simulink model "PIDController"  (R2025b)
settings: Solver=FixedStepAuto  StartTime=0.0  StopTime=inf  FixedStep=.002  RelTol=1e-3
libraries: simulink x3
settings Model: Creator=ajax  LastModifiedBy=ajax

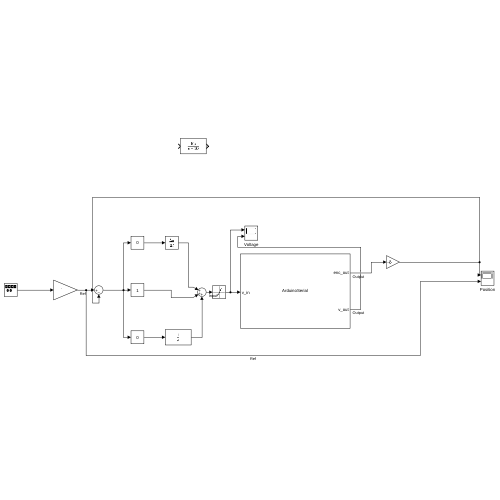
[thumbnail: Simulink's stored preview of the top-level diagram]
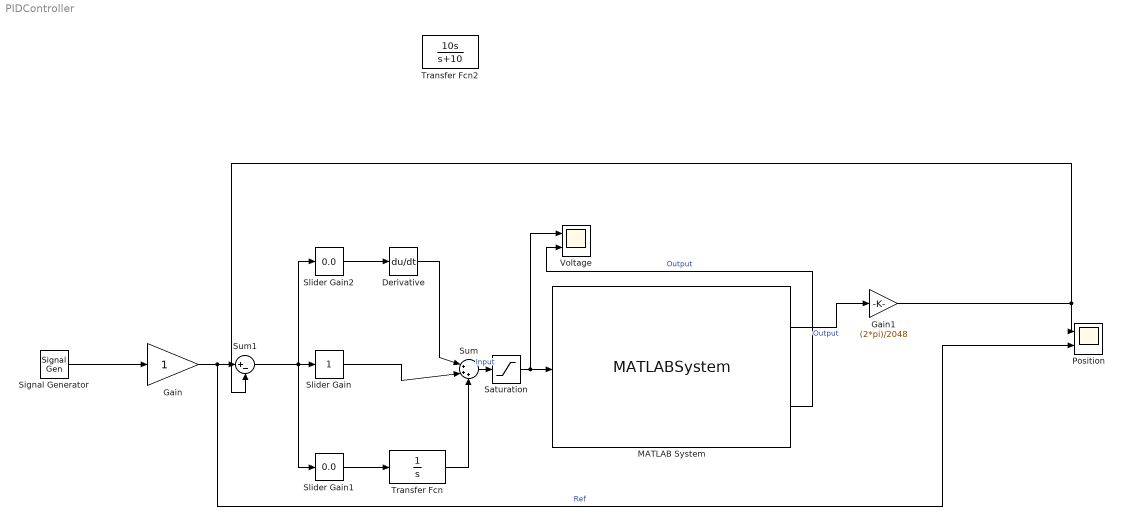
== system PIDController ==
  Derivative : Derivative
  Gain : Gain
  Gain1 : Gain  Gain=(2*pi)/2048
  MATLAB System : MATLABSystem  System=ArduinoSerial  COMPort=/dev/ttyACM0  BaudRate=115200  TimerPeriod=0.005  SimulateUsing=Interpreted execution
      mask Type: ArduinoSerial
  Position : Scope  NumInputPorts=2
      settings: ActiveDisplayYMinimum=-365.02359945676773  ActiveDisplayYMaximum=873.0296356104534
  Saturation : Saturate  UpperLimit=3  LowerLimit=-3
  Signal Generator : SignalGenerator  WaveForm=square  Frequency=.5
  Slider Gain : simulink/Math Operations/Slider Gain  gain=1  low=0  high=2
  Slider Gain1 : simulink/Math Operations/Slider Gain  gain=0.0  low=0  high=2
  Slider Gain2 : simulink/Math Operations/Slider Gain  gain=0.0  low=0  high=10
  Sum : Sum  Inputs=|+++
  Sum1 : Sum  Inputs=|+-
  Transfer Fcn : TransferFcn  Denominator=[1 0]
  Transfer Fcn2 : TransferFcn  Numerator=[10 0]  Denominator=[1 10]
  Voltage : Scope  NumInputPorts=2
      settings: ActiveDisplayYMinimum=-7.1806488970151925  ActiveDisplayYMaximum=7.8345844750588949
  wires:
  Slider Gain/1 -> Sum/2
  Slider Gain1/1 -> Transfer Fcn/1
  Transfer Fcn/1 -> Sum/3
  MATLAB System/1 -> Gain1/1  "Output"
  Gain/1 -> Position/2, Sum1/1  "Ref"
  MATLAB System/2 -> Voltage/2  "Output"
  Sum1/1 -> Slider Gain2/1, Slider Gain1/1, Slider Gain/1
  Gain1/1 -> Sum1/2, Position/1
  Sum/1 -> Saturation/1  "Input"
  Saturation/1 -> Voltage/1, MATLAB System/1
  Signal Generator/1 -> Gain/1
  Slider Gain2/1 -> Derivative/1
  Derivative/1 -> Sum/1
